simulink model "anM"  (R2018a)
settings: Solver=VariableStepAuto  StartTime=0.0  StopTime=10.0  RelTol=1e-3
settings Model: Creator=Катя  LastModifiedBy=Катя

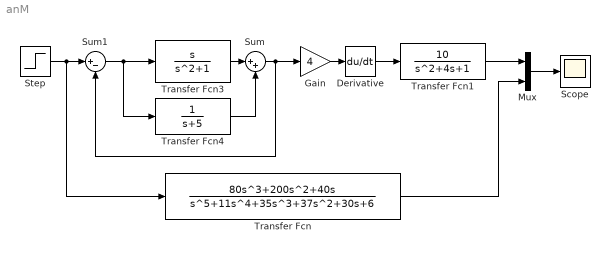
== system anM ==
  Derivative : Derivative
  Gain : Gain  Gain=4
  Mux : Mux  Inputs=2
  Scope : Scope
  Step : Step  Time=0  SampleTime=0
  Sum : Sum  Inputs=|++
  Sum1 : Sum  Inputs=|+-
  Transfer Fcn : TransferFcn  Numerator=[80 200 40 0]  Denominator=[1 11 35 37 30 6]
  Transfer Fcn1 : TransferFcn  Numerator=[10]  Denominator=[1 4 1]
  Transfer Fcn3 : TransferFcn  Numerator=[1 0]  Denominator=[1 0 1]
  Transfer Fcn4 : TransferFcn  Denominator=[1 5]
  wires:
  Sum1/1 -> Transfer Fcn4/1, Transfer Fcn3/1
  Transfer Fcn3/1 -> Sum/1
  Transfer Fcn4/1 -> Sum/2
  Sum/1 -> Gain/1, Sum1/2
  Derivative/1 -> Transfer Fcn1/1
  Transfer Fcn1/1 -> Mux/1
  Transfer Fcn/1 -> Mux/2
  Mux/1 -> Scope/1
  Step/1 -> Transfer Fcn/1, Sum1/1
  Gain/1 -> Derivative/1
